simulink model "PID_2RD_TEST"  (Simulink 7.6)
settings: Solver=ode45  StartTime=0.0  StopTime=20  RelTol=1e-3
settings Model: Creator=Administrator  LastModifiedBy=Administrator
settings DebuggingCC: AlgebraicLoopMsg=none  ArtificialAlgebraicLoopMsg=none  SolverPrmCheckMsg=none  UnknownTsInhSupMsg=none

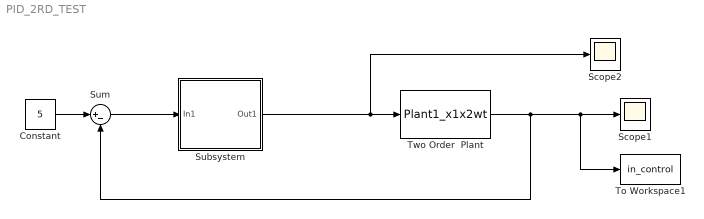
== system PID_2RD_TEST ==
  Constant : Constant  Value=5
  Scope1 : Scope
      settings: TimeRange=30  YMin=5  YMax=5.0003  DataFormat=Array
  Scope2 : Scope
      settings: TimeRange=200  YMin=0  YMax=500  DataFormat=Array
  Subsystem : Subsystem  mask{P=20, I=5, D=0, S=0}
      mask prompts: P "proporation"; I "integrator"; D "derivative"; S "antigain"
      mask Display: disp('SPID\nControl')
  Sum : Sum  Inputs=|+-
  To Workspace1 : ToWorkspace  VariableName=in_control  SampleTime=1  SaveFormat=Array
  Two Order  Plant : S-Function  FunctionName=Plant1_x1x2wt  EnableBusSupport=off
  wires:
  Two Order  Plant/1 -> Sum/2, Scope1/1, To Workspace1/1
  Subsystem/1(Out1) -> Two Order  Plant/1, Scope2/1
  Constant/1 -> Sum/1
  Sum/1 -> Subsystem/1(In1)

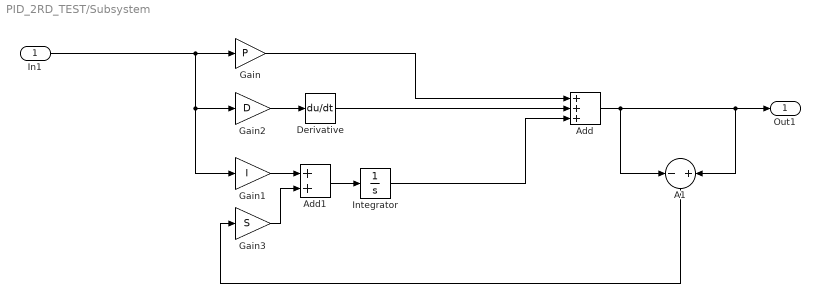
== system PID_2RD_TEST/Subsystem ==
  In1 : Inport
  A1 : Sum  Inputs=-+
  Add : Sum  Inputs=+++
  Add1 : Sum
  Derivative : Derivative
  Gain : Gain  Gain=P
  Gain1 : Gain  Gain=I
  Gain2 : Gain  Gain=D
  Gain3 : Gain  Gain=S
  Integrator : Integrator
  Out1 : Outport
  wires:
  In1/1 -> Gain/1, Gain2/1, Gain1/1
  Gain/1 -> Add/1
  Gain2/1 -> Derivative/1
  Add/1 -> A1/1, Out1/1, A1/2
  Derivative/1 -> Add/2
  Integrator/1 -> Add/3
  A1/1 -> Gain3/1
  Gain1/1 -> Add1/1
  Add1/1 -> Integrator/1
  Gain3/1 -> Add1/2
